simulink model "AdvancedWork"  (R2024b)
settings: Solver=VariableStepAuto  StartTime=0.0  StopTime=40  RelTol=1e-3
libraries: robotsim3dlib x1, sim3dlib x1
settings Model: Creator=dd217  LastModifiedBy=dd217

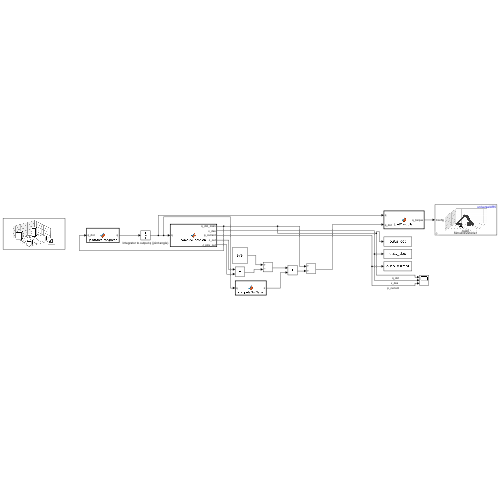
[thumbnail: Simulink's stored preview of the top-level diagram]
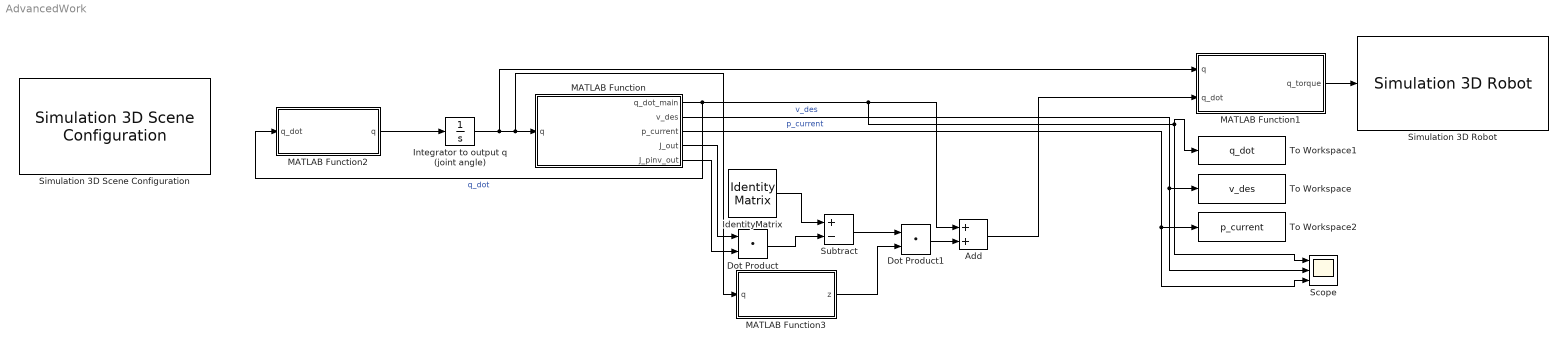
== system AdvancedWork ==
  Add : Sum
  Dot Product : DotProduct  OutDataTypeStr=Inherit: Inherit via internal rule
  Dot Product1 : DotProduct  OutDataTypeStr=Inherit: Inherit via internal rule
  IdentityMatrix : IdentityMatrix  OutputDimensions=2
  Integrator to output q (joint angle) : Integrator
  MATLAB Function : MATLAB Function  TreatAsAtomicUnit=on  SystemSampleTime=0.01
  MATLAB Function1 : MATLAB Function  TreatAsAtomicUnit=on  SystemSampleTime=0.01
  MATLAB Function2 : MATLAB Function  TreatAsAtomicUnit=on  SystemSampleTime=0.01
  MATLAB Function3 : MATLAB Function  TreatAsAtomicUnit=on
  Scope : Scope  NumInputPorts=3
  Simulation 3D Robot : robotsim3dlib/Simulation 3D Robot  actorInputType=Robot Library  RigidBodyTree=universalUR5  ActorName=SimulinkVehicle1  existActorChekBox=off  initialTrans=[0 0 0]  initialRot=[0 0 0]  initialConfig="[0  0  0  0  0  0]"  EndEffector=tool0  eeOffsetInpChekBox=off  eeTargetTrans=[0 0 0]  eeTargetRot=[0 0 0]  enableRegionGraspChekBox=off  regionGraspInpChekBox=off  eeTargTransDiff=[0.2 0.2 0.2]  eeTargRotDiff=[0 0 0]  inpConfEnbVal=on  inpGraspEnbVal=off  inpTransEnbVal=off  outConfEnbVal=off  outGraspEnbVal=off  outTransEnbVal=off  SampleTime=0.01  ActorType=SimulinkVehicle  ID=1  aMode=6  ActorTag=SimulinkVehicle1  Mesh=RigidBodyTree
  Simulation 3D Scene Configuration : sim3dlib/Simulation 3D Scene Configuration  Priority=-1  ProjectFormat=Default Scenes  SceneDesc=Empty scene  ProjectName=C:\Program Files\MATLAB\R2024b\toolbox\shared\sim3d_projects\automotive_project_windows\UE\WindowsNoEditor\VehicleSimulation.exe  ScenePath=/Game/Maps/EmptyScene  EnableOpenDRIVE=off  vehTagList={'<empty>';'Scene Origin';'SimulinkVehicle1'}  vehTag=Scene Origin  FreeCameraInitialTranslation=[0, 0, 0]  FreeCameraDefaultInitialTranslation=[-6, 0, 2]  FreeCameraInitialRotation=[0, 0, 0]  FreeCameraDefaultInitialRotation=[0, -15, 0]  OpVisEn=off  Ts=0.01  EnableWindow=on  EnableRemoteAccess=off  EnableWeather=off  SunAzimuth=90  SunAltitude=40.0  EnableGeospatialSun=off  Latitude=0  Longitude=0  Date=2023-01-01  Time=10:30:00  GeoTimeZone=-5.0  SunDaylightSaving=off  wind=1  clouds=10  EnableVolumetricClouds=off  CloudCoverage=0  CloudAltitude=6  fog=0  rain=0  RaindropsEffect=off  SnowDensity=0  EnableGeospatial=off  UseTrueOrigin=off  OriginHeight=200  OriginLatitude=40.744652  OriginLongitude=-73.988864  MapStyle=Aerial  AdditionalAssetIDs=[]  UseAdvancedSunSky=off  SolarTime=11  TimeZone=-5  Day=21  Month=9  Year=2022  UseDaylightSavingTime=on  DSTStartDay=10  DSTStartMonth=3  DSTEndDay=3  DSTEndMonth=11  DSTSwitchHour=2  sensorTag=MainCamera1  sensorId=1  sensorName=MainCamera1  mountLoc=Origin  offsetFlag=off  tmountOffset=[0, 0, 0]  rmountOffset=[0, 0, 0]  HorizontalResolution=1280  VerticalResolution=720  HorizontalFOV=60  mountPoint=[0 0 0]  mountOrientation=[0 0 0]  aMode=6  ID=1  GeoTrigger=Inactive
      settings: LibrarySourceBlock=robotsim3dlib/Simulation 3D Scene Configuration
  Subtract : Sum  Inputs=+-
  To Workspace : ToWorkspace  VariableName=v_des  SaveFormat=Structure With Time  SampleTime=0.01
      settings: Save2DSignal=2-D array (concatenate along first dimension)
  To Workspace1 : ToWorkspace  VariableName=q_dot  SaveFormat=Structure With Time  SampleTime=0.01
      settings: Save2DSignal=2-D array (concatenate along first dimension)
  To Workspace2 : ToWorkspace  VariableName=p_current  SaveFormat=Structure With Time  SampleTime=0.01
      settings: Save2DSignal=2-D array (concatenate along first dimension)
  wires:
  MATLAB Function/3(p_current) -> Scope/3, To Workspace2/1  "p_current"
  Integrator to output q (joint angle)/1 -> MATLAB Function1/1(q), MATLAB Function3/1(q), MATLAB Function/1(q)
  MATLAB Function1/1(q_torque) -> Simulation 3D Robot/1
  MATLAB Function/1(q_dot_main) -> MATLAB Function2/1(q_dot), Add/1, To Workspace1/1, Scope/1  "q_dot"
  MATLAB Function2/1(q) -> Integrator to output q (joint angle)/1
  MATLAB Function/2(v_des) -> Scope/2, To Workspace/1  "v_des"
  MATLAB Function/4(J_out) -> Dot Product/1
  MATLAB Function/5(J_pinv_out) -> Dot Product/2
  IdentityMatrix/1 -> Subtract/1
  Dot Product/1 -> Subtract/2
  Subtract/1 -> Dot Product1/1
  MATLAB Function3/1(z) -> Dot Product1/2
  Dot Product1/1 -> Add/2
  Add/1 -> MATLAB Function1/2(q_dot)

== matlab function AdvancedWork/MATLAB Function1 ==
  data: q input; q_torque output; q_dot input
function q_torque = jointController(q, q_dot)
Kp = 5;% Proportional gain
Kd = 0.3; % Differential gain

% PD control output
q_torque = -Kp * q - Kd *q_dot;

end

== matlab function AdvancedWork/MATLAB Function ==
  data: q input; q_dot_main output; v_des output; p_current output; J_out output; J_pinv_out output
function [q_dot_main, v_des, p_current, J_out, J_pinv_out] = computeJacobian(q)

% Declare extrinsic functions
coder.extrinsic('geometricJacobian');
coder.extrinsic('getTransform');
coder.extrinsic('loadrobot');

% Initialize outputs
q_dot = zeros(6,1);
v_des = zeros(6,1);
p_current = zeros(3,1);

% Load robot model
robot = loadrobot('universalUR5', 'DataFormat', 'column');

% Compute Jacobian
J = geometricJacobian(robot, q, 'tool0');
J = double(J);
rank(J)

% % Check condition number instead of rank
% if cond(J) > 1e10
%     warning('Jacobian is ill-conditioned. Skipping update.');
%     return;
% end

% Compute Jacobian pseudoinverse
J_pinv = pinv(J);

% Desired position
%p_des = [0.5; 0.2; 0.3];
%p_des = [0.3; 0.2; 0.2]; 
p_des = [0.2; 0.1; 0.3];

% Get current position
T = getTransform(robot, q, 'tool0');
T = double(T);
p_current = T(1:3, 4);

% Compute position error
e = p_des - p_current;

% Gain
Kp = 0.18;
v_des_linear = Kp * e;
v_des = [v_des_linear; zeros(3,1)];

% Stopping condition
if norm(e) < 0.01
    v_des = zeros(6,1);
end

% Compute q_dot with fault tolerance
q_dot_temp = J_pinv * v_des;

% Fault tolerance
if any(isnan(q_dot_temp)) || any(isinf(q_dot_temp))
    q_dot = zeros(6,1);
else
    q_dot = q_dot_temp;
end

% Smooth joint velocity limit
q_dot = 0.5 * tanh(q_dot / 0.5);  % Limit each joint velocity to [-0.5, 0.5]

% Compute Jacobian
J = geometricJacobian(robot, q, 'tool0');
J = double(J);
J_pinv = pinv(J);

% Main project speed
q_dot_main = J_pinv * v_des;

% Output original Jacobian
J_out = J;
J_pinv_out = J_pinv;


end

== matlab function AdvancedWork/MATLAB Function2 ==
  data: q_dot input; q output
% function q = jointStateIntegrator(q_dot)
% %#codegen
% persistent q_prev;
% if isempty(q_prev)
%     % Initial joint angles
%     q_prev = [0; -pi/2; pi/2; 0; pi/4; 0];
% end
% 
% % Set sample time (should match Simulink model)
% Ts = 0.01;
% 
% % Euler integration
% q = q_prev + Ts * q_dot;
% 
% % To prevent the abnormal q
% if any(isnan(q)) || any(isinf(q))
%     q = q_prev;  % q = zeros(6,1);
% end
% 
% 
% 
% % Update state
% q_prev = q;


function q = jointStateIntegrator(q_dot)
%#codegen

persistent q_prev;
if isempty(q_prev)
    % Initial joint angles
    q_prev = [0; -pi/3; pi/2; 0; pi/3; 0];
end

% Sample time
Ts = 0.01;

% Euler integration
q = q_prev + Ts * q_dot;

% Limit the joint angle to the physical range
q_min = [-pi; -pi; -pi; -pi; -pi; -pi];
q_max = [ pi;  pi;  pi;  pi;  pi;  pi];
q = min(max(q, q_min), q_max);  % Limit q to the range [q_min, q_max]

% Prevent NaN / Inf explosion
if any(isnan(q)) || any(isinf(q))
    q = q_prev;
end

% Update memory
q_prev = q;

== matlab function AdvancedWork/MATLAB Function3 ==
  data: q input; z output
function z = computeNullTerm(q)
    %#codegen
    q_center = [0; 0; 0; 0; 0; 0];
    gain = 0.1;
    z = -gain * (q - q_center);
end
